simulink model "sampleModel7293_pp_1_1_mu"  (R2018a)
settings: Solver=VariableStepAuto  StartTime=0.0  StopTime=10.0  RelTol=1e-3
undefined symbols (not defined in the file): DiscIntNeverNeededParam
libraries: simulink x367
(part 13 of 13)

== system sampleModel7293_pp_1_1_mu/cfblk209/cfblk9/cfblk17 ==
  emi_122 : Inport
  Action Port : ActionPort  ActionType=then
  cfblk17 : Delay
  emi_123 : Outport
  wires:
  emi_122/1 -> cfblk17/1
  cfblk17/1 -> emi_123/1

== system sampleModel7293_pp_1_1_mu/cfblk209/cfblk9/cfblk4 ==
  emi_1230 : Inport
  Action Port : ActionPort  ActionType=then
  cfblk4 : simulink/Discrete/Transfer Fcn First Order  PoleZ=0.95  ICPrevOutput=0.0  DoSatur=off
      settings: SourceProductName=Simulink
  emi_1231 : Outport
  wires:
  emi_1230/1 -> cfblk4/1
  cfblk4/1 -> emi_1231/1

== system sampleModel7293_pp_1_1_mu/cfblk209/cfblk9/emi_1232 ==
  Action Port : ActionPort  ActionType=else
  emi_1233 : Assertion

== system sampleModel7293_pp_1_1_mu/cfblk209/cfblk9/emi_124 ==
  Action Port : ActionPort  ActionType=else
  emi_125 : Assertion

== system sampleModel7293_pp_1_1_mu/cfblk209/cfblk9/emi_1901 ==
  Action Port : ActionPort  ActionType=else
  emi_1902 : Assertion

== system sampleModel7293_pp_1_1_mu/cfblk210/cfblk18/cfblk4 ==
  emi_1579 : Inport
  Action Port : ActionPort  ActionType=then
  cfblk4 : simulink/Continuous/PID Controller  Controller=PID  TimeDomain=Discrete-time  SampleTime=-1  IntegratorMethod=Forward Euler  FilterMethod=Forward Euler  Form=Parallel  UseFilter=on  ControllerParametersSource=internal  P=1  I=1  D=0  N=100  InitialConditionSource=internal  InitialConditionForIntegrator=0  InitialConditionForFilter=0  ExternalReset=none  LimitOutput=off  UpperSaturationLimit=inf  LowerSaturationLimit=-inf  LinearizeAsGain=off  AntiWindupMode=none  Kb=1  TrackingMode=off  Kt=1  PParamMin=[]  PParamMax=[]  IParamMin=[]  IParamMax=[]  DParamMin=[]  DParamMax=[]  NParamMin=[]  NParamMax=[]  KbParamMin=[]  KbParamMax=[]  KtParamMin=[]  KtParamMax=[]  POutMin=[]  POutMax=[]  IOutMin=[]  IOutMax=[]  DOutMin=[]  DOutMax=[]  NOutMin=[]  NOutMax=[]  KbOutMin=[]  KbOutMax=[]  KtOutMin=[]  KtOutMax=[]  IntegratorOutMin=[]  IntegratorOutMax=[]  FilterOutMin=[]  FilterOutMax=[]  SumOutMin=[]  SumOutMax=[]  SumI1OutMin=[]  SumI1OutMax=[]  SumI2OutMin=[]  SumI2OutMax=[]  SumI3OutMin=[]  SumI3OutMax=[]  SumDOutMin=[]  SumDOutMax=[]  SaturationOutMin=[]  SaturationOutMax=[]  IntegratorContinuousStateAttributes=''  IntegratorStateMustResolveToSignalObject=off  IntegratorRTWStateStorageClass=Auto  FilterContinuousStateAttributes=''  FilterStateMustResolveToSignalObject=off  FilterRTWStateStorageClass=Auto  DifferentiatorICPrevScaledInput=0  DifferentiatorOutMin=[]  DifferentiatorOutMax=[]  FilterDiffOutCoefMin=[]  FilterDiffOutCoefMax=[]  SumDenOutMin=[]  SumDenOutMax=[]  SumNumOutMin=[]  SumNumOutMax=[]  ReciprocalOutMin=[]  ReciprocalOutMax=[]  DivideOutMin=[]  DivideOutMax=[]  TunerSelectOption=Transfer Function Based (PID Tuner App)
  emi_1580 : Outport
  wires:
  emi_1579/1 -> cfblk4/1
  cfblk4/1 -> emi_1580/1

== system sampleModel7293_pp_1_1_mu/cfblk210/cfblk18/cfblk9 ==
  emi_1686 : Inport
  Action Port : ActionPort  ActionType=then
  cfblk9 : simulink/Discrete/Transfer Fcn Lead or Lag  PoleZ=0.95  ZeroZ=0.75  ICPrevOutput=0.0  ICPrevInput=0.0  DoSatur=off
      settings: SourceProductName=Simulink  SourceProductBaseCode=SL
  emi_1687 : Outport
  wires:
  emi_1686/1 -> cfblk9/1
  cfblk9/1 -> emi_1687/1

== system sampleModel7293_pp_1_1_mu/cfblk210/cfblk18/emi_1581 ==
  Action Port : ActionPort  ActionType=else
  emi_1582 : Assertion

== system sampleModel7293_pp_1_1_mu/cfblk210/cfblk18/emi_1688 ==
  Action Port : ActionPort  ActionType=else
  emi_1689 : Assertion

== system sampleModel7293_pp_1_1_mu/cfblk213/cfblk14/cfblk12 ==
  emi_552 : Inport
  emi_553 : Inport  Port=2
  Action Port : ActionPort  ActionType=then
  cfblk12 : Delay  DelayLengthSource=Input port
      settings: InputPortMap=u0,p1
  emi_554 : Outport
  wires:
  emi_552/1 -> cfblk12/1
  emi_553/1 -> cfblk12/2
  cfblk12/1 -> emi_554/1

== system sampleModel7293_pp_1_1_mu/cfblk213/cfblk14/cfblk16 ==
  emi_795 : Inport
  Action Port : ActionPort  ActionType=then
  cfblk16 : Delay
  emi_796 : Outport
  wires:
  emi_795/1 -> cfblk16/1
  cfblk16/1 -> emi_796/1

== system sampleModel7293_pp_1_1_mu/cfblk213/cfblk14/cfblk17 ==
  emi_1100 : Inport
  Action Port : ActionPort  ActionType=then
  cfblk17 : Delay
  emi_1101 : Outport
  wires:
  emi_1100/1 -> cfblk17/1
  cfblk17/1 -> emi_1101/1

== system sampleModel7293_pp_1_1_mu/cfblk213/cfblk14/cfblk19 ==
  emi_29 : Inport
  Action Port : ActionPort  ActionType=then
  cfblk19 : DataTypeConversion  OutDataTypeStr=double
  emi_30 : Outport
  wires:
  emi_29/1 -> cfblk19/1
  cfblk19/1 -> emi_30/1

== system sampleModel7293_pp_1_1_mu/cfblk213/cfblk14/cfblk6 ==
  emi_588 : Inport
  emi_589 : Inport  Port=2
  Action Port : ActionPort  ActionType=then
  cfblk6 : Delay  ShowEnablePort=on
      settings: InputPortMap=u0,e6
  emi_590 : Outport
  wires:
  emi_588/1 -> cfblk6/1
  emi_589/1 -> cfblk6/2
  cfblk6/1 -> emi_590/1

== system sampleModel7293_pp_1_1_mu/cfblk213/cfblk14/emi_1102 ==
  Action Port : ActionPort  ActionType=else
  emi_1103 : Assertion

== system sampleModel7293_pp_1_1_mu/cfblk213/cfblk14/emi_31 ==
  Action Port : ActionPort  ActionType=else
  emi_32 : Assertion

== system sampleModel7293_pp_1_1_mu/cfblk213/cfblk14/emi_555 ==
  Action Port : ActionPort  ActionType=else
  emi_556 : Assertion

== system sampleModel7293_pp_1_1_mu/cfblk213/cfblk14/emi_591 ==
  Action Port : ActionPort  ActionType=else
  emi_592 : Assertion

== system sampleModel7293_pp_1_1_mu/cfblk213/cfblk14/emi_797 ==
  Action Port : ActionPort  ActionType=else
  emi_798 : Assertion
